simulink model "Suspension_derivative_example"  (R2017b)
settings: Solver=VariableStepAuto  StartTime=0.0  StopTime=91  RelTol=1e-3
settings Model: Creator=mm395  LastModifiedBy=mm395

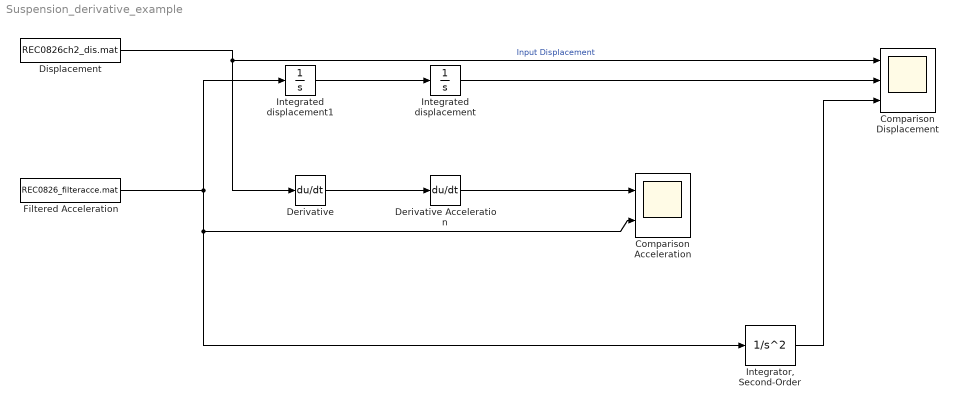
== system Suspension_derivative_example ==
  Comparison Acceleration : Scope  NumInputPorts=2
  Comparison Displacement : Scope  NumInputPorts=3
  Derivative : Derivative  CoefficientInTFapproximation=0
  Derivative Acceleration : Derivative  CoefficientInTFapproximation=0
  Displacement : FromFile  FileName=REC0826ch2_dis.mat  SampleTime=1/3200  ExtrapolationBeforeFirstDataPoint=Hold first value  ExtrapolationAfterLastDataPoint=Hold last value
  Filtered Acceleration : FromFile  FileName=REC0826_filteracce.mat  SampleTime=1/3200  ExtrapolationBeforeFirstDataPoint=Hold first value  ExtrapolationAfterLastDataPoint=Hold last value
  Integrated displacement : Integrator
  Integrated displacement1 : Integrator
  "Integrator, Second-Order" : SecondOrderIntegrator  ShowOutput=x
  wires:
  Integrated displacement/1 -> Comparison Displacement/2
  Integrated displacement1/1 -> Integrated displacement/1
  Displacement/1 -> Derivative/1, Comparison Displacement/1  "Input Displacement"
  Filtered Acceleration/1 -> "Integrator, Second-Order"/1, Comparison Acceleration/2, Integrated displacement1/1
  Derivative/1 -> Derivative Acceleration/1
  Derivative Acceleration/1 -> Comparison Acceleration/1
  "Integrator, Second-Order"/1 -> Comparison Displacement/3
